simulink model "Sistema_de_control_de_posicion 2"  (R2019a)
settings: Solver=VariableStepAuto  StartTime=0.0  StopTime=10.0  RelTol=1e-3
undefined symbols (not defined in the file): DiscIntNeverNeededParam, error_margin, refx, refy, Ts, w0, x0, y0
libraries: simulink x1
settings Model: Creator=mrblissfulgrin  LastModifiedBy=mrblissfulgrin

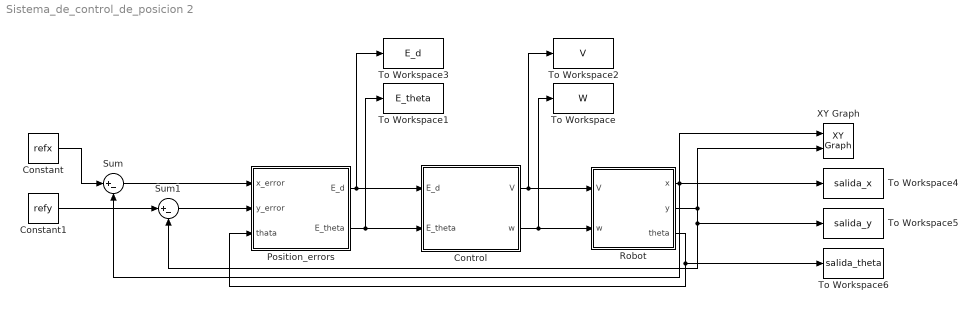
== system Sistema_de_control_de_posicion 2 ==
  Constant : Constant  Value=refx  SampleTime=Ts
  Constant1 : Constant  Value=refy  SampleTime=Ts
  Control : Subsystem
  Position_errors : Subsystem
  Robot : Subsystem
  Sum : Sum  Inputs=|+-
  Sum1 : Sum  Inputs=|+-
  To Workspace : ToWorkspace  VariableName=W  SaveFormat=Structure With Time  SampleTime=Ts
  To Workspace1 : ToWorkspace  VariableName=E_theta  SaveFormat=Structure With Time  SampleTime=Ts
  To Workspace2 : ToWorkspace  VariableName=V  SaveFormat=Structure With Time  SampleTime=Ts
  To Workspace3 : ToWorkspace  VariableName=E_d  SaveFormat=Structure With Time  SampleTime=Ts
  To Workspace4 : ToWorkspace  VariableName=salida_x  SaveFormat=Structure With Time  SampleTime=Ts
  To Workspace5 : ToWorkspace  VariableName=salida_y  SaveFormat=Structure With Time  SampleTime=Ts
  To Workspace6 : ToWorkspace  VariableName=salida_theta  SaveFormat=Structure With Time  SampleTime=Ts
  XY Graph : simulink/Sinks/XY Graph  xmin=-10  xmax=10  ymin=-10  ymax=10  st=Ts
  wires:
  Control/1(V) -> To Workspace2/1, Robot/1(V)
  Control/2(w) -> To Workspace/1, Robot/2(w)
  Position_errors/1(E_d) -> To Workspace3/1, Control/1(E_d)
  Position_errors/2(E_theta) -> To Workspace1/1, Control/2(E_theta)
  Robot/2(y) -> To Workspace5/1, Sum1/2, XY Graph/2
  Robot/3(theta) -> To Workspace6/1, Position_errors/3(thata)
  Robot/1(x) -> XY Graph/1, To Workspace4/1, Sum/2
  Sum/1 -> Position_errors/1(x_error)
  Sum1/1 -> Position_errors/2(y_error)
  Constant/1 -> Sum/1
  Constant1/1 -> Sum1/1

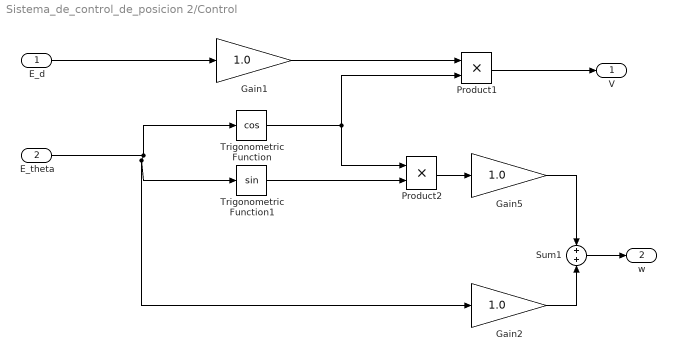
== system Sistema_de_control_de_posicion 2/Control ==
  E_d : Inport
  E_theta : Inport  Port=2
  Gain1 : Gain  Gain=1.0
  Gain2 : Gain  Gain=1.0
  Gain5 : Gain  Gain=1.0
  Product1 : Product
  Product2 : Product
  Sum1 : Sum
  Trigonometric Function : Trigonometry  Operator=cos
  Trigonometric Function1 : Trigonometry
  V : Outport
  w : Outport  Port=2
  wires:
  E_theta/1 -> Trigonometric Function/1, Trigonometric Function1/1, Gain2/1
  E_d/1 -> Gain1/1
  Trigonometric Function/1 -> Product1/2, Product2/1
  Product1/1 -> V/1
  Trigonometric Function1/1 -> Product2/2
  Product2/1 -> Gain5/1
  Gain1/1 -> Product1/1
  Gain5/1 -> Sum1/1
  Gain2/1 -> Sum1/2
  Sum1/1 -> w/1

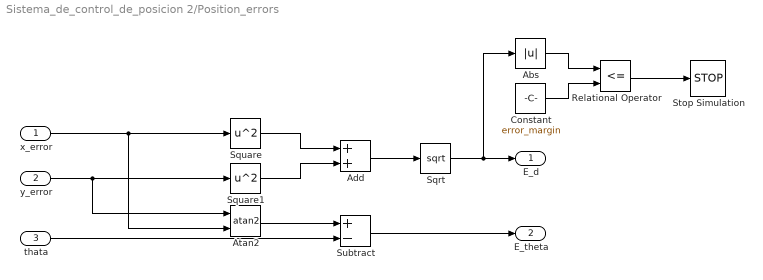
== system Sistema_de_control_de_posicion 2/Position_errors ==
  x_error : Inport  SampleTime=Ts
  y_error : Inport  Port=2  SampleTime=Ts
  thata : Inport  Port=3  SampleTime=Ts
  Abs : Abs
  Add : Sum
  Atan2 : Trigonometry  Operator=atan2
  Constant : Constant  Value=error_margin  SampleTime=Ts
  Relational Operator : RelationalOperator  Operator=<=  OutDataTypeStr=boolean  RndMeth=Simplest
  Sqrt : Sqrt  SaturateOnIntegerOverflow=on
  Square : Math  Operator=square  SaturateOnIntegerOverflow=on
  Square1 : Math  Operator=square  SaturateOnIntegerOverflow=on
  Stop Simulation : Stop
  Subtract : Sum  Inputs=+-
  E_d : Outport  SampleTime=Ts
  E_theta : Outport  Port=2  SampleTime=Ts
  wires:
  Square/1 -> Add/1
  Atan2/1 -> Subtract/1
  Sqrt/1 -> E_d/1, Abs/1
  y_error/1 -> Square1/1, Atan2/1
  Add/1 -> Sqrt/1
  Square1/1 -> Add/2
  thata/1 -> Subtract/2
  x_error/1 -> Square/1, Atan2/2
  Subtract/1 -> E_theta/1
  Abs/1 -> Relational Operator/1
  Constant/1 -> Relational Operator/2
  Relational Operator/1 -> Stop Simulation/1

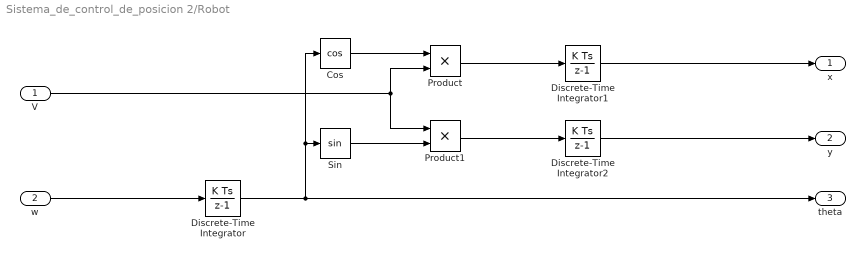
== system Sistema_de_control_de_posicion 2/Robot ==
  V : Inport  SampleTime=Ts
  w : Inport  Port=2  SampleTime=Ts
  Cos : Trigonometry  Operator=cos
  Discrete-Time Integrator : DiscreteIntegrator  InitialCondition=w0  SampleTime=Ts  ICPrevOutput=DiscIntNeverNeededParam  ICPrevScaledInput=DiscIntNeverNeededParam
  Discrete-Time Integrator1 : DiscreteIntegrator  InitialCondition=x0  SampleTime=Ts  ICPrevOutput=DiscIntNeverNeededParam  ICPrevScaledInput=DiscIntNeverNeededParam
  Discrete-Time Integrator2 : DiscreteIntegrator  InitialCondition=y0  SampleTime=Ts  ICPrevOutput=DiscIntNeverNeededParam  ICPrevScaledInput=DiscIntNeverNeededParam
  Product : Product
  Product1 : Product
  Sin : Trigonometry
  x : Outport  SampleTime=Ts
  y : Outport  Port=2  SampleTime=Ts
  theta : Outport  Port=3  SampleTime=Ts
  wires:
  Discrete-Time Integrator2/1 -> y/1
  Product1/1 -> Discrete-Time Integrator2/1
  Cos/1 -> Product/1
  Sin/1 -> Product1/2
  w/1 -> Discrete-Time Integrator/1
  Discrete-Time Integrator1/1 -> x/1
  Product/1 -> Discrete-Time Integrator1/1
  V/1 -> Product/2, Product1/1
  Discrete-Time Integrator/1 -> theta/1, Sin/1, Cos/1
